simulink model "clamped_plate_KIRCHHOFF_FEM_aug"  (R2025b)
settings: Solver=VariableStepAuto  StartTime=0.0  StopTime=10  RelTol=1e-3
libraries: RCTblocks x1
settings Model: Creator=f.sanfedino  LastModifiedBy=andre
settings SolverCC: AlgebraicLoopSolver=TrustRegion
settings DataIOCC: ReturnWorkspaceOutputs=off
settings DebuggingCC: UnconnectedInputMsg=warning  UnconnectedOutputMsg=warning  UnconnectedLineMsg=warning
settings ModelReferenceCC: EnableRefExpFcnMdlSchedulingChecks=on
settings RTWCC: GPUComputeCapability=3.5  DLArmComputeVersion=19.05

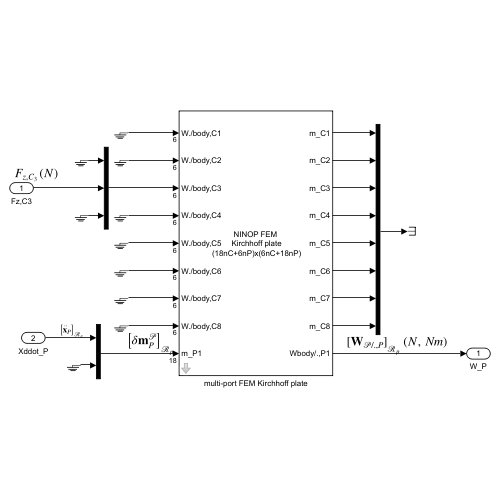
[thumbnail: Simulink's stored preview of the top-level diagram]
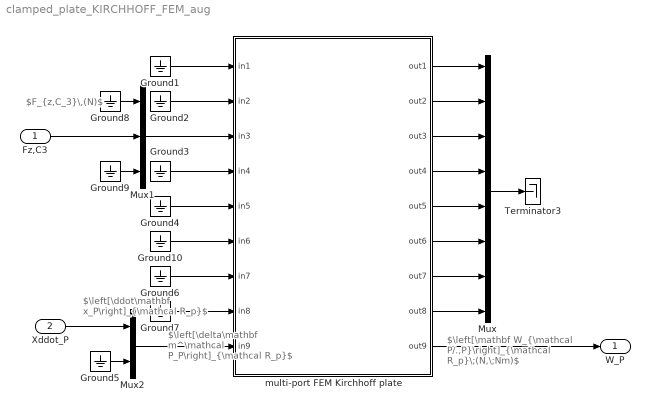
== system clamped_plate_KIRCHHOFF_FEM_aug ==
  note: $F_{z,C_3}\,(N)$
  note: $\left[\mathbf W_{\mathcal P/.,P}\right]_{\mathcal R_p}\;(N,\;Nm)$
  note: $\left[\delta\mathbf m^\mathcal P_P\right]_{\mathcal R_p}$
  note: $\left[\ddot\mathbf x_P\right]_{\mathcal R_p}$
  Fz,C3 : Inport
  Xddot_P : Inport  Port=2
  Ground{1..10} (10 alike) : Ground
  Mux : Mux  Inputs=18*ones(1,8)
  Mux1 : Mux  Inputs=[2 1 3]
  Mux2 : Mux  Inputs=[6 12]
  Terminator3 : Terminator
  multi-port FEM Kirchhoff plate : Subsystem  mask(Multi-port flexible plate (18nC+6nP)x(6nC+18nP)){lx=1, ly=1, t=0.003, rho=2015.8, E=69.87e9, ni=0.5764, xi=0.001, nx=10, ny=10, i_nP=1, i_nC=8, P1=56, P2=20, P3=25, P4=20, C1=1, C2=6, C3=11, C4=61, C5=66, C6=111, C7=116, C8=121, RedSlowOn=off, RedFastOn=on, w_trunc=1000, uw_var=0, Nflex=0}
      mask prompts: lx "lenght along x (m)"; ly "length along y (m)"; t "thickness (m)"; rho "mass density (Kg/m^3)"; E "Young modulus (N/m^2)"; ni "Poisson coefficient"; xi "damping coefficient"; nx "number of elements along x (integer)"; ny "number of elements along y (integer)"; i_nP "number (nP) of parent (P) nodes (<5)"; i_nC "number (nC) of child (C) nodes"; P1 "P1 (integer)"; P2 "P2 (integer)"; P3 "P3 (integer)"; P4 "P4 (integer)"; C1 "C1 (integer)"; C2 "C2 (integer)"; C3 "C3 (integer)"; C4 "C4 (integer)"; C5 "C5 (integer)"; C6 "C6 (integer)"; C7 "C7 (integer)"; C8 "C8 (inreger)"; RedSlowOn "Reduction of the 6*(nP-1) poles at 0 (due to loop closure constraints when nP>1)."; RedFastOn "Reduction of fast flexible modes:"; w_trunc "with a frequency (rad/s) >"; uw_var "uncertainty (%)"; Nflex "number of flexible modes (Nf, integer)"
      mask help:
      | (18nC+6nP)x(6nC+18nP) multi-port model of a uniform plate (in the x-y plane) between
      |   *  wrenches applied to the plate at the given nC child nodes (input) and motion vectors at these child nodes (output)
      |   *  motion vectors at the nP parent nodes (input)  and wrenches applied by this plate at these parent nodes (output)
      |  dynamic model of a uniform flexible plate (in the x-y plane),
      | in the plate reference frame (0,x,y,z)
      |
      | The plate is defined by:
      | * 0<x<lx
      | * 0<y<ly
      | * -t/2<z<t/2
      |
      | This model is based on a finite element apprach using (nx x ny) elements (nx and ny elements along x and y axes, respectiveley).  The parents and child nodes must be specified by their indexes in the list of the (nx+1)x(n
      | y+1) nodes defined by:
      |  * node 1 is the point (0,0) of the plate,
      |  * node nx+1 is the point (lx,0) of the plate,
      |  * node nx+2 is the point (0, ly/ny) of the plate,
      |  * node 2*(nx+1) is the point (lx,ly/ny) of the plate,
      |  * ....
      |  * node j*(nx+1) is the point (lx,(j-1)*ly/ny) of the plate,
      |  * node j*(nx+1)+1 is the point (0, j*ly/ny) of the plate,
      |  * ...
      |  * node (ny+1)*(nx+1) is the point (lx,ly) of the plate.
      |
      | This block can also performed optional model reductions:
      |    * reduction of the 6*(nP-1) poles at 0 due to loop closure constraints,
      |    * reduction of the flexible modes which a frequnecy (rad/s) greated than a specified value.
      |
      | See the inline help for more details.
      |
      | All parameters are expressed in the plate reference fram.
      | Dynamics in translations along x and y and rotation around z are assumed rigid.
      mask init:
      | MultiPortFEMKirchhoffPlateAug
      mask Help: web('DocPlate_Kirchhoff.html','-browser')
      mask TypeOptions i_nP: 0 | 1 | 2 | 3 | 4
      mask TypeOptions i_nC: 0 | 1 | 2 | 3 | 4 | 5 | 6 | 7 | 8
      mask DialogControl ParameterGroupVar Prompt: Main parameters
      mask DialogControl Pport1 Prompt: P node #1
      mask DialogControl Pport2 Prompt: #2
      mask DialogControl Pport3 Prompt: #3
      mask DialogControl Pport4 Prompt: #4
      mask DialogControl Cport1 Prompt: C node #1
      mask DialogControl Cport2 Prompt: #2
      mask DialogControl Cport3 Prompt: #3
      mask DialogControl Cport4 Prompt: #4
      mask DialogControl Cport5 Prompt: #5
      mask DialogControl Cport6 Prompt: #6
      mask DialogControl Cport7 Prompt: #7
      mask DialogControl Cport8 Prompt: #8
      mask DialogControl Reduction Prompt: Optional Reduction
      mask DialogControl Container21 Prompt: Parametric uncertainties
      mask DialogControl Control2 Prompt: The uncertain parameters are the first Nf cantilevered frequencies of the plate when it is clamped at the first parent node (P1) or the last child node CnC when the number of parent nodes is null.
      mask DialogControl Control3 Prompt: The uncertain frequency is named: 'w_name_i' where:
      mask DialogControl Control4 Prompt: * 'name' is the current block name (reduced to its alphanumeric characters).
      mask DialogControl Control5 Prompt: * 'i' is the flexible mode number (increasing frequency order)
      mask Display:
      | disp('NINOP FEM\n Kirchhoff plate\n (18nC+6nP)x(6nC+18nP)')
      | if nC~=0
      |     for ii=1:nC
      |         port_label('input', ii, ['W./body,C',num2str(ii)])
      |         port_label('output',ii,['m_C',num2str(ii)])
      |     end
      | end
      | if nP~=0
      |     for ii=1:nP
      |         port_label('input', nC+ii, ['m_P',num2str(ii)])
      |         port_label('output',nC+ii,['Wbody/.,P',num2str(ii)])
      |     end
      | end
  W_P : Outport
  wires:
  Mux2/1 -> multi-port FEM Kirchhoff plate/9(in9)
  Ground1/1 -> multi-port FEM Kirchhoff plate/1(in1)
  Ground2/1 -> multi-port FEM Kirchhoff plate/2(in2)
  Ground4/1 -> multi-port FEM Kirchhoff plate/5(in5)
  Ground3/1 -> multi-port FEM Kirchhoff plate/4(in4)
  Ground6/1 -> multi-port FEM Kirchhoff plate/7(in7)
  Ground7/1 -> multi-port FEM Kirchhoff plate/8(in8)
  multi-port FEM Kirchhoff plate/1(out1) -> Mux/1
  multi-port FEM Kirchhoff plate/2(out2) -> Mux/2
  multi-port FEM Kirchhoff plate/3(out3) -> Mux/3
  multi-port FEM Kirchhoff plate/4(out4) -> Mux/4
  multi-port FEM Kirchhoff plate/5(out5) -> Mux/5
  multi-port FEM Kirchhoff plate/6(out6) -> Mux/6
  multi-port FEM Kirchhoff plate/7(out7) -> Mux/7
  multi-port FEM Kirchhoff plate/8(out8) -> Mux/8
  multi-port FEM Kirchhoff plate/9(out9) -> W_P/1
  Mux1/1 -> multi-port FEM Kirchhoff plate/3(in3)
  Ground8/1 -> Mux1/1
  Ground9/1 -> Mux1/3
  Ground10/1 -> multi-port FEM Kirchhoff plate/6(in6)
  Fz,C3/1 -> Mux1/2
  Mux/1 -> Terminator3/1
  Xddot_P/1 -> Mux2/1
  Ground5/1 -> Mux2/2

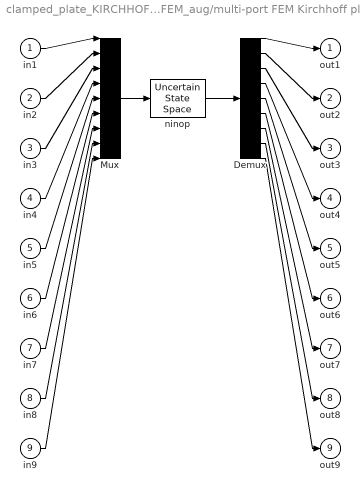
== system clamped_plate_KIRCHHOFF_FEM_aug/multi-port FEM Kirchhoff plate ==
  in1 : Inport  PortDimensions=6
  in2 : Inport  Port=2  PortDimensions=6
  in3 : Inport  Port=3  PortDimensions=6
  in4 : Inport  Port=4  PortDimensions=6
  in5 : Inport  Port=5  PortDimensions=6
  in6 : Inport  Port=6  PortDimensions=6
  in7 : Inport  Port=7  PortDimensions=6
  in8 : Inport  Port=8  PortDimensions=6
  in9 : Inport  Port=9  PortDimensions=18
  Demux : Demux  Outputs=[18 18 18 18 18 18 18 18 6 ]
  Mux : Mux  Inputs=[6 6 6 6 6 6 6 6 18 ]
  ninop : RCTblocks/Uncertain State Space  Tag=USS  USystem=NINOP  UValue=[]  X0=[]  uX0=[]
  out1 : Outport
  out2 : Outport  Port=2
  out3 : Outport  Port=3
  out4 : Outport  Port=4
  out5 : Outport  Port=5
  out6 : Outport  Port=6
  out7 : Outport  Port=7
  out8 : Outport  Port=8
  out9 : Outport  Port=9
  wires:
  Mux/1 -> ninop/1
  ninop/1 -> Demux/1
  in1/1 -> Mux/1
  Demux/1 -> out1/1
  in2/1 -> Mux/2
  Demux/2 -> out2/1
  in3/1 -> Mux/3
  Demux/3 -> out3/1
  in4/1 -> Mux/4
  Demux/4 -> out4/1
  in5/1 -> Mux/5
  Demux/5 -> out5/1
  in6/1 -> Mux/6
  Demux/6 -> out6/1
  in7/1 -> Mux/7
  Demux/7 -> out7/1
  in8/1 -> Mux/8
  Demux/8 -> out8/1
  in9/1 -> Mux/9
  Demux/9 -> out9/1
